simulink model "IQ_To_PL"  (R2018b)
settings: Solver=VariableStepAuto  StartTime=0.0  StopTime=(128*1024*100)*10e-9  RelTol=1e-3
libraries: xbsIndex_r4 x35
settings Model: SimulationMode=accelerator  Creator=marsiau  LastModifiedBy=marsiau

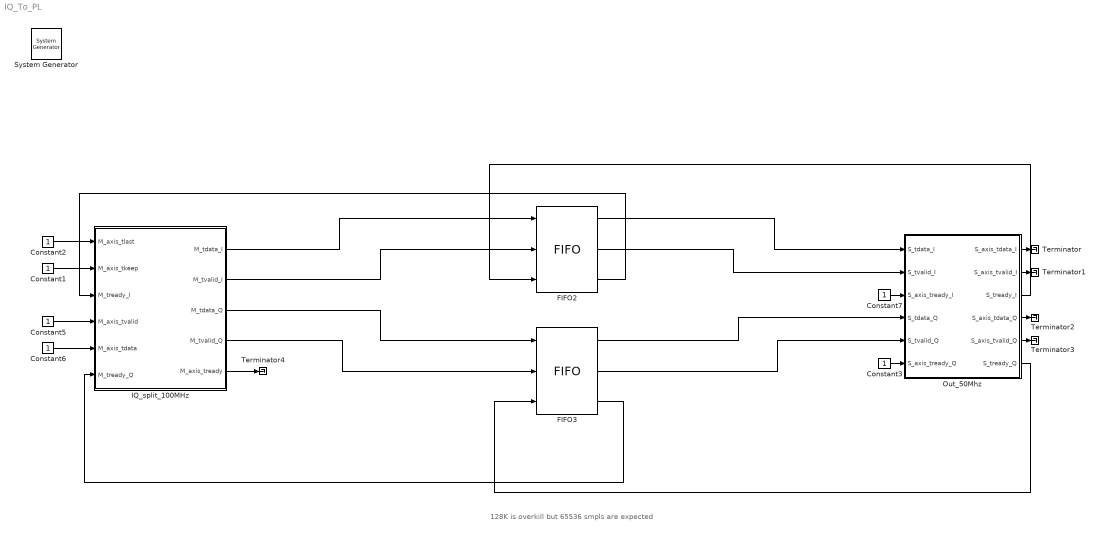
== system IQ_To_PL ==
  note: 128K is overkill but 65536 smpls are expected
  " System Generator" : xbsIndex_r4/ System Generator  Tag=genX  xilinxfamily=zynq  part=xc7z020  speed=-1  package=clg400  synthesis_tool=Vivado  clock_wrapper=Clock Enables  directory=./netlist  proj_type=Vivado  Synth_file=Vivado Synthesis Defaults  Impl_file=Vivado Implementation Defaults  testbench=off  simulink_period=1  sysclk_period=10  dcm_input_clock_period=10  incr_netlist=off  trim_vbits=Everywhere in SubSystem  dbl_ovrd=According to Block Masks  core_generation=According to Block Masks  run_coregen=off  deprecated_control=off  eval_field=0  block_type=sysgen
  Constant{1..3,5..7} (6 alike) : Constant  OutDataTypeStr=boolean  SampleTime=10e-9
  FIFO2 : xbsIndex_r4/FIFO  mem_type=Block RAM  performance_options=Standard_FIFO  embedded_registers=off  depth=128K  percent_nbits=1  rst=off  rst_latency=1  en=off  use_dcount=off  use_percent_full_port=off  use_almost_empty=off  almost_empty_thresh=2  use_almost_full=off  almost_full_thresh=14  explicit_period=off  dbl_ovrd=off  block_type=fifo
  FIFO3 : xbsIndex_r4/FIFO  mem_type=Block RAM  performance_options=Standard_FIFO  embedded_registers=off  depth=128K  percent_nbits=1  rst=off  rst_latency=1  en=off  use_dcount=off  use_percent_full_port=off  use_almost_empty=off  almost_empty_thresh=2  use_almost_full=off  almost_full_thresh=14  explicit_period=off  dbl_ovrd=off  block_type=fifo
  IQ_split_100MHz : Subsystem
  Out_50Mhz : Subsystem
  Terminator{,1..4} (5 alike) : Terminator
  wires:
  Out_50Mhz/6(S_tready_Q) -> FIFO3/3
  IQ_split_100MHz/4(M_tvalid_Q) -> FIFO3/2
  FIFO2/1 -> Out_50Mhz/1(S_tdata_I)
  Constant3/1 -> Out_50Mhz/6(S_axis_tready_Q)
  Constant6/1 -> IQ_split_100MHz/5(M_axis_tdata)
  Out_50Mhz/4(S_axis_tdata_Q) -> Terminator2/1
  IQ_split_100MHz/2(M_tvalid_I) -> FIFO2/2
  FIFO2/3 -> IQ_split_100MHz/3(M_tready_I)
  Constant7/1 -> Out_50Mhz/3(S_axis_tready_I)
  IQ_split_100MHz/1(M_tdata_I) -> FIFO2/1
  Constant2/1 -> IQ_split_100MHz/1(M_axis_tlast)
  FIFO3/2 -> Out_50Mhz/5(S_tvalid_Q)
  Constant1/1 -> IQ_split_100MHz/2("M_axis_tkeep ")
  Constant5/1 -> IQ_split_100MHz/4(M_axis_tvalid)
  FIFO3/3 -> IQ_split_100MHz/6(M_tready_Q)
  FIFO2/2 -> Out_50Mhz/2(S_tvalid_I)
  FIFO3/1 -> Out_50Mhz/4(S_tdata_Q)
  Out_50Mhz/1(S_axis_tdata_I) -> Terminator/1
  IQ_split_100MHz/3(M_tdata_Q) -> FIFO3/1
  IQ_split_100MHz/5(M_axis_tready) -> Terminator4/1
  Out_50Mhz/5(S_axis_tvalid_Q) -> Terminator3/1
  Out_50Mhz/3(S_tready_I) -> FIFO2/3
  Out_50Mhz/2(S_axis_tvalid_I) -> Terminator1/1

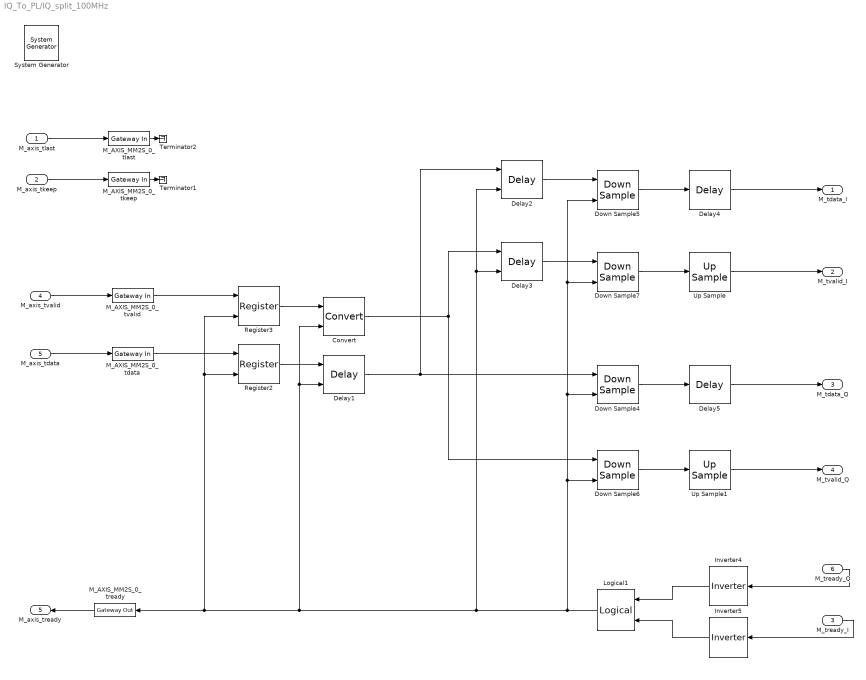
== system IQ_To_PL/IQ_split_100MHz ==
  M_axis_tlast : Inport
  "M_axis_tkeep " : Inport  Port=2
  M_tready_I : Inport  Port=3
  M_axis_tvalid : Inport  Port=4
  M_axis_tdata : Inport  Port=5
  M_tready_Q : Inport  Port=6
  " System Generator" : xbsIndex_r4/ System Generator  Tag=genX  xilinxfamily=zynq  part=xc7z020  speed=-1  package=clg400  synthesis_tool=Vivado  clock_wrapper=Clock Enables  directory=./netlist  proj_type=Vivado  Synth_file=Vivado Synthesis Defaults  Impl_file=Vivado Implementation Defaults  testbench=off  simulink_period=10e-9  sysclk_period=10  dcm_input_clock_period=10  incr_netlist=off  trim_vbits=Everywhere in SubSystem  dbl_ovrd=According to Block Masks  core_generation=According to Block Masks  run_coregen=off  deprecated_control=off  eval_field=0  block_type=sysgen
  Convert : xbsIndex_r4/Convert  gui_display_data_type=Boolean  arith_type=Boolean  n_bits=16  bin_pt=14  float_type=Single  exp_bits=8  fraction_bits=24  quantization=Truncate  overflow=Wrap  en=on  latency=1  pipeline=off  dbl_ovrd=off  block_type=convert
  Delay1 : xbsIndex_r4/Delay  rst=off  infoeditControl=Selection of Reset will increase slice count due to use of real FFs and instead of SRLs  en=on  latency=1  reg_retiming=off  dbl_ovrd=off  block_type=delay
  Delay2 : xbsIndex_r4/Delay  rst=off  infoeditControl=Selection of Reset will increase slice count due to use of real FFs and instead of SRLs  en=on  latency=1  reg_retiming=off  dbl_ovrd=off  block_type=delay
  Delay3 : xbsIndex_r4/Delay  rst=off  infoeditControl=Selection of Reset will increase slice count due to use of real FFs and instead of SRLs  en=on  latency=1  reg_retiming=off  dbl_ovrd=off  block_type=delay
  Delay4 : xbsIndex_r4/Delay  rst=off  infoeditControl=Selection of Reset will increase slice count due to use of real FFs and instead of SRLs  en=off  latency=1  reg_retiming=off  dbl_ovrd=off  block_type=delay
  Delay5 : xbsIndex_r4/Delay  rst=off  infoeditControl=Selection of Reset will increase slice count due to use of real FFs and instead of SRLs  en=off  latency=1  reg_retiming=off  dbl_ovrd=off  block_type=delay
  Down Sample{4..7} (4 alike) : xbsIndex_r4/Down Sample  sample_ratio=2  sample_phase="Last Value of Frame  (most efficient)"  en=on  rst=off  latency=1  dbl_ovrd=off  block_type=dsamp
  Inverter4 : xbsIndex_r4/Inverter  en=off  latency=1  dbl_ovrd=off  block_type=inv
  Inverter5 : xbsIndex_r4/Inverter  en=off  latency=1  dbl_ovrd=off  block_type=inv
  Logical1 : xbsIndex_r4/Logical  logical_function=AND  inputs=2  en=off  latency=1  precision=Full  arith_type=Unsigned  n_bits=16  bin_pt=0  align_bp=on  dbl_ovrd=off  block_type=logical
  M_AXIS_MM2S_0_tdata : xbsIndex_r4/Gateway In  gui_display_data_type=Fixed-point  arith_type=Unsigned  n_bits=8  bin_pt=0  preci_type=Single  exp_width=8  frac_width=24  rows=1  columns=1  quantization="Round  (unbiased: +/- Inf)"  overflow=Saturate  period=10e-9  UseAsADC=off  ADCChannel='1'  interface=None  automatic_assignment=on  address_offset=hex2dec('00')  intf_name=''  intf_description=''  default_value=0  timing_constraint=None  locs_specified=off  LOCs={}  io_standard={}  inherit_from_input=off  hdl_port=on  dbl_ovrd=off  block_type=gatewayin
  M_AXIS_MM2S_0_tkeep : xbsIndex_r4/Gateway In  gui_display_data_type=Fixed-point  arith_type=Unsigned  n_bits=1  bin_pt=0  preci_type=Single  exp_width=8  frac_width=24  rows=1  columns=1  quantization="Round  (unbiased: +/- Inf)"  overflow=Saturate  period=10e-9  UseAsADC=off  ADCChannel='1'  interface=None  automatic_assignment=on  address_offset=hex2dec('00')  intf_name=''  intf_description=''  default_value=0  timing_constraint=None  locs_specified=off  LOCs={}  io_standard={}  inherit_from_input=off  hdl_port=on  dbl_ovrd=off  block_type=gatewayin
  M_AXIS_MM2S_0_tlast : xbsIndex_r4/Gateway In  gui_display_data_type=Fixed-point  arith_type=Unsigned  n_bits=1  bin_pt=0  preci_type=Single  exp_width=8  frac_width=24  rows=1  columns=1  quantization="Round  (unbiased: +/- Inf)"  overflow=Saturate  period=10e-9  UseAsADC=off  ADCChannel='1'  interface=None  automatic_assignment=on  address_offset=hex2dec('00')  intf_name=''  intf_description=''  default_value=0  timing_constraint=None  locs_specified=off  LOCs={}  io_standard={}  inherit_from_input=off  hdl_port=on  dbl_ovrd=off  block_type=gatewayin
  M_AXIS_MM2S_0_tready : xbsIndex_r4/Gateway Out  inherit_from_input=off  hdl_port=on  rows=1  columns=1  UseAsDAC=off  DACChannel='1'  interface=None  automatic_assignment=on  address_offset=hex2dec('00')  intf_name=''  intf_description=''  timing_constraint=None  locs_specified=off  LOCs={}  io_standard={}  block_type=gatewayout
  M_AXIS_MM2S_0_tvalid : xbsIndex_r4/Gateway In  gui_display_data_type=Fixed-point  arith_type=Unsigned  n_bits=1  bin_pt=0  preci_type=Single  exp_width=8  frac_width=24  rows=1  columns=1  quantization="Round  (unbiased: +/- Inf)"  overflow=Saturate  period=10e-9  UseAsADC=off  ADCChannel='1'  interface=None  automatic_assignment=on  address_offset=hex2dec('00')  intf_name=''  intf_description=''  default_value=0  timing_constraint=None  locs_specified=off  LOCs={}  io_standard={}  inherit_from_input=off  hdl_port=on  dbl_ovrd=off  block_type=gatewayin
  Register2 : xbsIndex_r4/Register  init=0  rst=off  en=on  dbl_ovrd=off  block_type=register
  Register3 : xbsIndex_r4/Register  init=0  rst=off  en=on  dbl_ovrd=off  block_type=register
  Terminator1 : Terminator
  Terminator2 : Terminator
  Up Sample : xbsIndex_r4/Up Sample  sample_ratio=2  copy_samples=off  en=off  latency=1  dbl_ovrd=off  block_type=usamp
  Up Sample1 : xbsIndex_r4/Up Sample  sample_ratio=2  copy_samples=off  en=off  latency=1  dbl_ovrd=off  block_type=usamp
  M_tdata_I : Outport
  M_tvalid_I : Outport  Port=2
  M_tdata_Q : Outport  Port=3
  M_tvalid_Q : Outport  Port=4
  M_axis_tready : Outport  Port=5
  wires:
  Up Sample1/1 -> M_tvalid_Q/1
  Inverter4/1 -> Logical1/1
  Delay5/1 -> M_tdata_Q/1
  M_AXIS_MM2S_0_tdata/1 -> Register2/1
  Delay2/1 -> Down Sample5/1
  M_AXIS_MM2S_0_tlast/1 -> Terminator2/1
  M_AXIS_MM2S_0_tready/1 -> M_axis_tready/1
  M_tready_Q/1 -> Inverter4/1
  M_AXIS_MM2S_0_tkeep/1 -> Terminator1/1
  M_tready_I/1 -> Inverter5/1
  M_axis_tvalid/1 -> M_AXIS_MM2S_0_tvalid/1
  "M_axis_tkeep "/1 -> M_AXIS_MM2S_0_tkeep/1
  Delay4/1 -> M_tdata_I/1
  Up Sample/1 -> M_tvalid_I/1
  Delay1/1 -> Delay2/1, Down Sample4/1
  M_axis_tdata/1 -> M_AXIS_MM2S_0_tdata/1
  Convert/1 -> Down Sample6/1, Delay3/1
  Inverter5/1 -> Logical1/2
  M_axis_tlast/1 -> M_AXIS_MM2S_0_tlast/1
  M_AXIS_MM2S_0_tvalid/1 -> Register3/1
  Delay3/1 -> Down Sample7/1
  Register2/1 -> Delay1/1
  Register3/1 -> Convert/1
  Logical1/1 -> Down Sample5/2, Down Sample7/2, Down Sample4/2, Down Sample6/2, Convert/2, Delay1/2, M_AXIS_MM2S_0_tready/1, Register3/2, Register2/2, Delay2/2, Delay3/2
  Down Sample5/1 -> Delay4/1
  Down Sample7/1 -> Up Sample/1
  Down Sample6/1 -> Up Sample1/1
  Down Sample4/1 -> Delay5/1

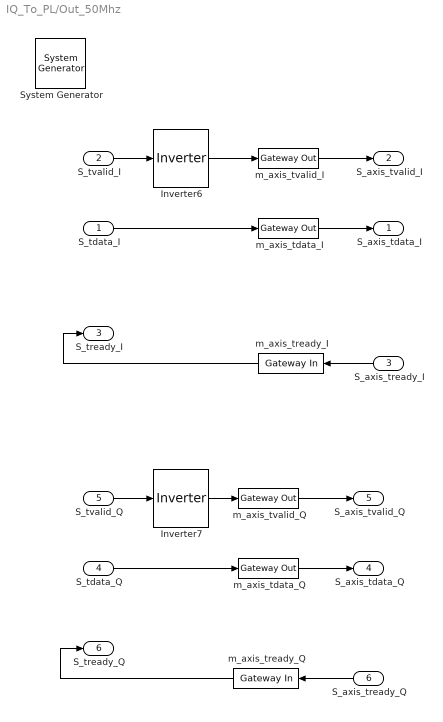
== system IQ_To_PL/Out_50Mhz ==
  S_tdata_I : Inport
  S_tvalid_I : Inport  Port=2
  S_axis_tready_I : Inport  Port=3  OutDataTypeStr=boolean
  S_tdata_Q : Inport  Port=4
  S_tvalid_Q : Inport  Port=5
  S_axis_tready_Q : Inport  Port=6  OutDataTypeStr=boolean
  " System Generator" : xbsIndex_r4/ System Generator  Tag=genX  xilinxfamily=zynq  part=xc7z020  speed=-1  package=clg400  synthesis_tool=Vivado  clock_wrapper=Clock Enables  directory=./netlist  proj_type=Vivado  Synth_file=Vivado Synthesis Defaults  Impl_file=Vivado Implementation Defaults  testbench=off  simulink_period=20e-9  sysclk_period=20  dcm_input_clock_period=10  incr_netlist=off  trim_vbits=Everywhere in SubSystem  dbl_ovrd=According to Block Masks  core_generation=According to Block Masks  run_coregen=off  deprecated_control=off  eval_field=0  block_type=sysgen
  Inverter6 : xbsIndex_r4/Inverter  en=off  latency=1  dbl_ovrd=off  block_type=inv
  Inverter7 : xbsIndex_r4/Inverter  en=off  latency=1  dbl_ovrd=off  block_type=inv
  m_axis_tdata_I : xbsIndex_r4/Gateway Out  inherit_from_input=on  hdl_port=on  rows=1  columns=1  UseAsDAC=off  DACChannel='1'  interface=None  automatic_assignment=on  address_offset=hex2dec('00')  intf_name=''  intf_description=''  timing_constraint=None  locs_specified=off  LOCs={}  io_standard={}  block_type=gatewayout
  m_axis_tdata_Q : xbsIndex_r4/Gateway Out  inherit_from_input=on  hdl_port=on  rows=1  columns=1  UseAsDAC=off  DACChannel='1'  interface=None  automatic_assignment=on  address_offset=hex2dec('00')  intf_name=''  intf_description=''  timing_constraint=None  locs_specified=off  LOCs={}  io_standard={}  block_type=gatewayout
  m_axis_tready_I : xbsIndex_r4/Gateway In  gui_display_data_type=Boolean  arith_type=Boolean  n_bits=16  bin_pt=14  preci_type=Single  exp_width=8  frac_width=24  rows=1  columns=1  quantization="Round  (unbiased: +/- Inf)"  overflow=Saturate  period=20e-9  UseAsADC=off  ADCChannel='1'  interface=None  automatic_assignment=on  address_offset=hex2dec('00')  intf_name=''  intf_description=''  default_value=0  timing_constraint=None  locs_specified=off  LOCs={}  io_standard={}  inherit_from_input=off  hdl_port=on  dbl_ovrd=off  block_type=gatewayin
  m_axis_tready_Q : xbsIndex_r4/Gateway In  gui_display_data_type=Boolean  arith_type=Boolean  n_bits=16  bin_pt=14  preci_type=Single  exp_width=8  frac_width=24  rows=1  columns=1  quantization="Round  (unbiased: +/- Inf)"  overflow=Saturate  period=20e-9  UseAsADC=off  ADCChannel='1'  interface=None  automatic_assignment=on  address_offset=hex2dec('00')  intf_name=''  intf_description=''  default_value=0  timing_constraint=None  locs_specified=off  LOCs={}  io_standard={}  inherit_from_input=off  hdl_port=on  dbl_ovrd=off  block_type=gatewayin
  m_axis_tvalid_I : xbsIndex_r4/Gateway Out  inherit_from_input=on  hdl_port=on  rows=1  columns=1  UseAsDAC=off  DACChannel='1'  interface=None  automatic_assignment=on  address_offset=hex2dec('00')  intf_name=''  intf_description=''  timing_constraint=None  locs_specified=off  LOCs={}  io_standard={}  block_type=gatewayout
  m_axis_tvalid_Q : xbsIndex_r4/Gateway Out  inherit_from_input=on  hdl_port=on  rows=1  columns=1  UseAsDAC=off  DACChannel='1'  interface=None  automatic_assignment=on  address_offset=hex2dec('00')  intf_name=''  intf_description=''  timing_constraint=None  locs_specified=off  LOCs={}  io_standard={}  block_type=gatewayout
  S_axis_tdata_I : Outport
  S_axis_tvalid_I : Outport  Port=2
  S_tready_I : Outport  Port=3
  S_axis_tdata_Q : Outport  Port=4
  S_axis_tvalid_Q : Outport  Port=5
  S_tready_Q : Outport  Port=6
  wires:
  S_axis_tready_Q/1 -> m_axis_tready_Q/1
  m_axis_tvalid_Q/1 -> S_axis_tvalid_Q/1
  S_tvalid_Q/1 -> Inverter7/1
  S_axis_tready_I/1 -> m_axis_tready_I/1
  S_tvalid_I/1 -> Inverter6/1
  m_axis_tvalid_I/1 -> S_axis_tvalid_I/1
  S_tdata_I/1 -> m_axis_tdata_I/1
  Inverter6/1 -> m_axis_tvalid_I/1
  m_axis_tdata_Q/1 -> S_axis_tdata_Q/1
  m_axis_tdata_I/1 -> S_axis_tdata_I/1
  m_axis_tready_I/1 -> S_tready_I/1
  S_tdata_Q/1 -> m_axis_tdata_Q/1
  Inverter7/1 -> m_axis_tvalid_Q/1
  m_axis_tready_Q/1 -> S_tready_Q/1
